simulink model "lab2_part2"  (R2023b)
settings: Solver=VariableStepAuto  StartTime=0.0  StopTime=30  RelTol=10e-10  AbsTol=10e-10
values from neighbouring files (symbols this model uses):
  A = [0, 1; 0, -alpha2/M]    [lab2.m]
  Actrl = A + B * K - L * C    [lab2.m]
  B = [0; alpha1/M]    [lab2.m]
  Bctrl = [L, -B * K]    [lab2.m]
  C = [1 0]    [lab2.m]
  Cctrl = K    [lab2.m]
  Dctrl = [0, -K]    [lab2.m]
settings Model: Creator=guxunjia  LastModifiedBy=markzhuang
settings SolverCC: AlgebraicLoopSolver=TrustRegion
settings DataIOCC: ReturnWorkspaceOutputs=off
settings DebuggingCC: UnconnectedInputMsg=warning  UnconnectedOutputMsg=warning  UnconnectedLineMsg=warning  ArithmeticOperatorsInVariantConditions=warning
settings ModelReferenceCC: EnableRefExpFcnMdlSchedulingChecks=on
settings SFSimCC: SimUseLocalCustomCode=off  CustomCodeUndefinedFunction=UseInterfaceOnly
settings RTWCC: RTWUseLocalCustomCode=off

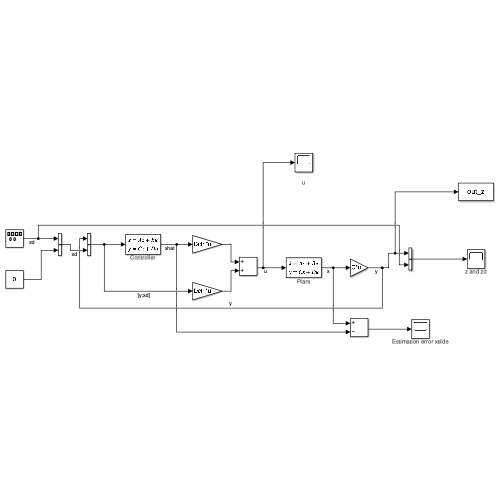
[thumbnail: Simulink's stored preview of the top-level diagram]
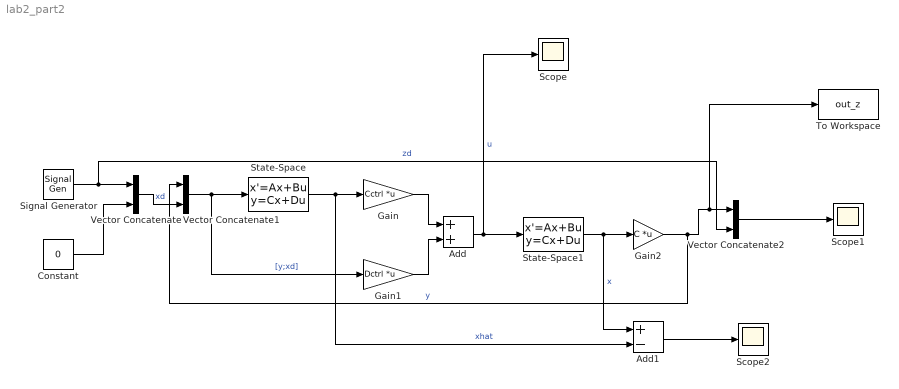
== system lab2_part2 ==
  Add : Sum
  Add1 : Sum  Inputs=+-
  Constant : Constant  Value=0
  Gain : Gain  Gain=Cctrl  Multiplication=Matrix(K*u)
  Gain1 : Gain  Gain=Dctrl  Multiplication=Matrix(K*u)
  Gain2 : Gain  Gain=C  Multiplication=Matrix(K*u)
  Scope : Scope
      settings: AttributesFormatString=u
  Scope1 : Scope
      settings: AttributesFormatString=z and zd
  Scope2 : Scope
      settings: AttributesFormatString=Estimation error xtilde
  Signal Generator : SignalGenerator  WaveForm=square  Amplitude=0.03  Frequency=0.1
  State-Space : StateSpace  A=Actrl  B=Bctrl  C=eye(2)  D=zeros(2,3)  InitialCondition=0
      settings: AttributesFormatString=Controller
  State-Space1 : StateSpace  A=A  B=B  C=eye(2)  D=zeros(2,1)  InitialCondition=0
      settings: AttributesFormatString=Plant
  To Workspace : ToWorkspace  VariableName=out_z  SaveFormat=Timeseries  SampleTime=-1
  Vector Concatenate : Concatenate
  Vector Concatenate1 : Concatenate
  Vector Concatenate2 : Concatenate
  wires:
  Signal Generator/1 -> Vector Concatenate2/2, Vector Concatenate/1  "zd"
  Constant/1 -> Vector Concatenate/2
  Vector Concatenate/1 -> Vector Concatenate1/2  "xd"
  Vector Concatenate1/1 -> Gain1/1, State-Space/1  "[y;xd]"
  State-Space/1 -> Add1/2, Gain/1  "xhat"
  Gain/1 -> Add/1
  Gain1/1 -> Add/2
  Add/1 -> State-Space1/1, Scope/1  "u"
  State-Space1/1 -> Add1/1, Gain2/1  "x"
  Gain2/1 -> Vector Concatenate1/1, To Workspace/1, Vector Concatenate2/1  "y"
  Vector Concatenate2/1 -> Scope1/1
  Add1/1 -> Scope2/1
